simulink model "nncACCsystem_5_50"  (R2021a)
(part 4 of 14)

  "IW{2,1}(50,:)'" : Constant  Value=[0.6144727511346823600746347437961958348751068115234375;-0.6043038220130103610472360742278397083282470703125;-0.783801644557404753044238532311283051967620849609375;0.3389010522781494838540083947009406983852386474609375;-0.58015357603872319547377855997183360159397125244140625;-0.0828531218332193564179988243267871439456939697265625;0.864527016971766926189957302995026111602783203125;-0.75405004236885975199555787185090593993663787841796875;-0.924872031665473937067645238130353391170501708984375;0.2032422703217200699032929378518019802868366241455078125;-0.51577685605288647874289154060534201562404632568359375;-0.4055467735335032131160915014334022998809814453125;0.05493671254072385323752314434386789798736572265625;0.67759451705134099430694050170131959021091461181640625;-0.4116803267880932981626074251835234463214874267578125;-0.47441335981344756600464052098686806857585906982421875;-0.2043561167782945720006182455108501017093658447265625;0.82617772384643439753659777124994434416294097900390625;0.67097567185446671533810558685217984020709991455078125;0.020372107650101778375528738251887261867523193359375;0.29447303762625243184203327473369427025318145751953125;0.9440215383879964061719647361314855515956878662109375;0.6089699130967947127146544517017900943756103515625;-0.374505969506301494842404053997597657144069671630859375;-0.317174623289982360319072540733031928539276123046875;-0.6531680775410075856513003600412048399448394775390625;-0.347181889319885417233280122673022560775279998779296875;-0.410264221687952901351792434070375747978687286376953125;0.8647688276796337003560211087460629642009735107421875;0.1110609867702390118893163162283599376678466796875;-0.9109852379156795354475661952164955437183380126953125;-0.563618771772022686405989588820375502109527587890625;0.92877626827141224197248448035679757595062255859375;0.7784042806215369925126879024901427328586578369140625;0.3473576102557089928524192146142013370990753173828125;0.5260876926599216130142622205312363803386688232421875;0.87918184720997538672548898830427788197994232177734375;-0.1541856848789065204119452801023726351559162139892578125;-0.8370901964404178219325558529817499220371246337890625;-0.1124822515347916607186817827823688276112079620361328125;0.6140848728942802647878806965309195220470428466796875;-0.10539002217157571184014130949435639195144176483154296875;-0.4184943899085287188910342592862434685230255126953125;0.80793144341254274909402965931803919374942779541015625;-0.8652517508433599235928568305098451673984527587890625;0.496355196733508474693508105701766908168792724609375;0.494053866935491026168847383814863860607147216796875;-0.56814383474823326736213857657276093959808349609375;-0.226886744375101923054671715362928807735443115234375;0.90268411668282910742533431402989663183689117431640625]
      mask Display: e = 0.06;c1 = [120 150 230]/255;c2 = ([120 150 230]+0)/383;c3 = ([120 150 230]+128)/383;patch([0 1 1 0],[0 0 1 1],c1);patch([0 1 1 1-e 1-e 0+e],[0 0 1 1-e 0+e 0+e],c2);patch([0 0 1 1-e 0+e 0+e],[0 1 1 1-e 1-e 0+e],c3);plot([0 1 1 0 0],[0 0 1 1 0]);disp('weights');
  "IW{2,1}(6,:)'" : Constant  Value=[0.9179696750633585811129933063057251274585723876953125;-0.88346646120579652716742202755995094776153564453125;0.244692976834197273294790875297621823847293853759765625;-0.9438452246350792496087933614035136997699737548828125;-0.51581422348284633461190651360084302723407745361328125;0.6392679962139224958406202858895994722843170166015625;0.39256092172291989772503484346088953316211700439453125;0.1274073475641765984534004019224084913730621337890625;0.983014382423863963822441291995346546173095703125;0.21261377652534430016117994455271400511264801025390625;-0.10676266904585872408173230496686301194131374359130859375;-0.1820218409406935133887373012839816510677337646484375;-0.9638203922685992797170229096082039177417755126953125;-0.2279018435819180343759882134690997190773487091064453125;0.6813804178287572455019471817649900913238525390625;-0.2319257096428964104450898275899817235767841339111328125;1.001130044802193364006370757124386727809906005859375;-0.040503476580812568241807269942000857554376125335693359375;-0.291956084314189345807477593552903272211551666259765625;-0.6641511544489426821513688992126844823360443115234375;0.18701086129516275580186857041553594172000885009765625;0.01889726273082524554691730145350447855889797210693359375;0.488466639896083132388326930595212616026401519775390625;-0.952184047085733453741340781562030315399169921875;-0.406201797611159154399729231954552233219146728515625;0.131173827637160567149976486689411103725433349609375;0.4246658792464617082629274591454304754734039306640625;0.030614624463881780214169481268982053734362125396728515625;-0.7653854213042341481099128941423259675502777099609375;0.492109159149804853417009553595562465488910675048828125;0.275738525125877043109312580781988799571990966796875;-0.5575165603951373061164531463873572647571563720703125;-0.2552990665415426629891726406640373170375823974609375;-0.446271264888553620409084032871760427951812744140625;-0.15871405452116960077546536922454833984375;-0.280849690565660115026958010275848209857940673828125;0.49259325590821223528337213792838156223297119140625;0.484247883080110186337918776189326308667659759521484375;0.91637163929900555814356266637332737445831298828125;0.72014198242155913476381101645529270172119140625;-0.26722753351259076470824993521091528236865997314453125;0.693474476935445949266068055294454097747802734375;0.06669875991181317687050977838225662708282470703125;-0.59487481996016289276241195693728514015674591064453125;0.193733150325572200944890255414065904915332794189453125;-0.6974229533286138149605903890915215015411376953125;-0.95023164977459229074696622774354182183742523193359375;-0.1834256124171742552420028005144558846950531005859375;-0.4783530129103301664628133949008770287036895751953125;-0.70751048127678106691718085130560211837291717529296875]
      mask Display: e = 0.06;c1 = [120 150 230]/255;c2 = ([120 150 230]+0)/383;c3 = ([120 150 230]+128)/383;patch([0 1 1 0],[0 0 1 1],c1);patch([0 1 1 1-e 1-e 0+e],[0 0 1 1-e 0+e 0+e],c2);patch([0 0 1 1-e 0+e 0+e],[0 1 1 1-e 1-e 0+e],c3);plot([0 1 1 0 0],[0 0 1 1 0]);disp('weights');
  "IW{2,1}(7,:)'" : Constant  Value=[-0.980867972090291306841436380636878311634063720703125;0.78971936348265792116052352866972796618938446044921875;0.039342120990233493682541876523828250356018543243408203125;0.3719800930434804531188319742796011269092559814453125;-0.595723059500692375678454482113011181354522705078125;-0.65476188012718683495450022746808826923370361328125;0.82079906581221118155866633969708345830440521240234375;0.78456959242778889773717310163192451000213623046875;0.1931230911806987027290460900985635817050933837890625;0.488427048366413651958595210089697502553462982177734375;0.05810490529781324464675407170943799428641796112060546875;0.438775605745484131858802356873638927936553955078125;0.6583963331479651959199372868170030415058135986328125;-0.143767182260148007610922604726511053740978240966796875;0.548926493081543842578184921876527369022369384765625;-0.256575387647672237267926220738445408642292022705078125;0.50717759017805530419309434364549815654754638671875;-0.8201705525611255875872984688612632453441619873046875;-0.81636875371478268004210576691548340022563934326171875;0.547756832701655316242295157280750572681427001953125;0.226396548255365870350175327985198237001895904541015625;-0.5050091514285259819416751270182430744171142578125;-0.376156424391524690786781093265744857490062713623046875;-0.483965229362445292782268779774312861263751983642578125;0.7671583652660542984591529602766968309879302978515625;-0.66759413476073614646111309411935508251190185546875;-0.149536285868914486929526219682884402573108673095703125;0.0356486383257654804168623741134069859981536865234375;-0.5364809912488761600712905419641174376010894775390625;0.379635766555958209522714241757057607173919677734375;-0.75807806746091888072669462417252361774444580078125;-0.8879521425628060793400209149695001542568206787109375;-0.001835753065937861805423381156288087368011474609375;0.4303370024846924213335341846686787903308868408203125;0.00830634558469700579053096589632332324981689453125;-0.4866911527767816547651591463363729417324066162109375;0.9410161792518543233398986558313481509685516357421875;0.6566193894160627930745022240444086492061614990234375;0.405020058591355702759528867318294942378997802734375;0.53907900563998001342014276815461926162242889404296875;-0.04110989433774604739912916784305707551538944244384765625;0.5029607066132768533606167693505994975566864013671875;-0.8955860226761480635815360074047930538654327392578125;0.490153693698361203612279268782003782689571380615234375;0.3058058094721205488752957535325549542903900146484375;-0.4447196145408434109214113050256855785846710205078125;-0.4646406314654412117448600838542915880680084228515625;-0.8677939966654582004679241435951553285121917724609375;0.275123247728420228241930090007372200489044189453125;-0.11899464474923256152028017140764859504997730255126953125]
      mask Display: e = 0.06;c1 = [120 150 230]/255;c2 = ([120 150 230]+0)/383;c3 = ([120 150 230]+128)/383;patch([0 1 1 0],[0 0 1 1],c1);patch([0 1 1 1-e 1-e 0+e],[0 0 1 1-e 0+e 0+e],c2);patch([0 0 1 1-e 0+e 0+e],[0 1 1 1-e 1-e 0+e],c3);plot([0 1 1 0 0],[0 0 1 1 0]);disp('weights');
  "IW{2,1}(8,:)'" : Constant  Value=[-0.06407735399410119381258255089051090180873870849609375;-0.68283082031059694205765708829858340322971343994140625;-0.6603161059148481282221609944826923310756683349609375;-0.3706914380762513783196254735230468213558197021484375;-0.73915158636827260618673562930780462920665740966796875;0.73428975350198388838407481671310961246490478515625;0.95060218635651538843234220621525309979915618896484375;-0.9067290700610886045041070246952585875988006591796875;-0.8332732167303802395252887436072342097759246826171875;0.9368319573378396381002630732837133109569549560546875;0.94557012232950043983947807646472938358783721923828125;-0.170516226437212647937258225283585488796234130859375;-0.545073815603446032440615454106591641902923583984375;0.465538414095752306476327930795378051698207855224609375;-0.81784853188574135884891802561469376087188720703125;-0.1544869675737840231111164257526979781687259674072265625;0.332258729184919332499958954940666444599628448486328125;0.37661552490315608476834086104645393788814544677734375;-0.9116536259519205653845119741163216531276702880859375;-0.4143449320257059920180608969531022012233734130859375;0.1009242949167486746997468571862555108964443206787109375;0.85027929850237427000791967657278291881084442138671875;-0.305503660416293898460793343474506400525569915771484375;0.4267785913559709598530389484949409961700439453125;-0.3730091636459429427219447461538948118686676025390625;0.9594325721361993686286950833164155483245849609375;-0.94925395456621297629595801481627859175205230712890625;-0.086621871321167276391861378215253353118896484375;-0.92117713836218317879911410273052752017974853515625;-0.9749126796252569615575112038641236722469329833984375;-0.9359913347500865565820049596368335187435150146484375;0.34944472215558874950147583149373531341552734375;0.9804309399166719618534671099041588604450225830078125;-0.702038840148247356154342924128286540508270263671875;-0.4831739393233416279826997197233140468597412109375;-0.13903125857727705039224019856192171573638916015625;0.1790054588197100560176266981216031126677989959716796875;-0.28130555663841316782480816982570104300975799560546875;-0.165029675175454304536515337531454861164093017578125;0.29762772429512096561410317008267156779766082763671875;0.07987012236004879806028355915259453468024730682373046875;0.147230642125261212971309987551649101078510284423828125;-0.59547301053531764836179718258790671825408935546875;-0.314192711422670967191805857510189525783061981201171875;-0.10479329307725386566385594733219477348029613494873046875;-0.494784453168344295903580132289789617061614990234375;0.84635061232047592572058647419908083975315093994140625;0.6462217446144540300423386725015006959438323974609375;-0.753402215742656977681690477766096591949462890625;-0.51731503262576661317240223070257343351840972900390625]
      mask Display: e = 0.06;c1 = [120 150 230]/255;c2 = ([120 150 230]+0)/383;c3 = ([120 150 230]+128)/383;patch([0 1 1 0],[0 0 1 1],c1);patch([0 1 1 1-e 1-e 0+e],[0 0 1 1-e 0+e 0+e],c2);patch([0 0 1 1-e 0+e 0+e],[0 1 1 1-e 1-e 0+e],c3);plot([0 1 1 0 0],[0 0 1 1 0]);disp('weights');
  "IW{2,1}(9,:)'" : Constant  Value=[-0.102714725663822559198479211772792041301727294921875;0.4368170165488063361181048094294965267181396484375;-0.51179821386116230996776721440255641937255859375;-0.787132888983194778376173417200334370136260986328125;-0.6590563544371967896751129956101067364215850830078125;0.0784485917003274746406304984702728688716888427734375;-0.7862631079594495364659678671159781515598297119140625;0.805272154985862353981929118162952363491058349609375;-0.4183870521965247224471795561839826405048370361328125;0.2439889456538122392004197536152787506580352783203125;-0.501606876311778027144328007125295698642730712890625;0.8303594512562797458343766265898011624813079833984375;-0.2557645626674929228983046414214186370372772216796875;0.0319540177471291375610462637268938124179840087890625;-0.6444998703933177974789714426151476800441741943359375;0.3866189078107942211914860308752395212650299072265625;0.91232573693869856157334652380086481571197509765625;0.571427116455696992858293015160597860813140869140625;-0.9689301839636759172691427011159248650074005126953125;-0.2074717539773345276188365460257045924663543701171875;0.4953012002888812492784609275986440479755401611328125;-0.2659602519525348096607331171981059014797210693359375;0.1714702338959359639858348600682802498340606689453125;0.449448527641817197064710853737778961658477783203125;0.7469316764358662208422856565448455512523651123046875;-0.04222883079584160981312379590235650539398193359375;0.960848497813605373352174865431152284145355224609375;0.8105326403854800076942410669289529323577880859375;0.4344707041244746381636332444031722843647003173828125;0.0714152851764093821174128606799058616161346435546875;-0.331011733793374229861683488707058131694793701171875;0.0242470574157973572937407880090177059173583984375;-0.60912441145073170645218851859681308269500732421875;-0.1507646675101452782286060028127394616603851318359375;0.9280407269415540394419394942815415561199188232421875;0.1478420865894018998432102307560853660106658935546875;0.572746574072698688695481905597262084484100341796875;-0.80497354396350839778051522444002330303192138671875;0.6750655125951308122012051171623170375823974609375;-0.2406190148984588272895734917256049811840057373046875;0.0853845073917802732665904841269366443157196044921875;-0.0019238695503458469460156265995465219020843505859375;-0.359935279909433969436349798343144357204437255859375;-0.5085445449720047417230261999065987765789031982421875;-0.662466683688774704563684281310997903347015380859375;-0.622816308705548937751927951467223465442657470703125;0.782043018155911706656979731633327901363372802734375;0.3763126465426847033768353867344558238983154296875;0.814751469791895832628370044403709471225738525390625;-0.3952772922938365685041617325623519718647003173828125]
      mask Display: e = 0.06;c1 = [120 150 230]/255;c2 = ([120 150 230]+0)/383;c3 = ([120 150 230]+128)/383;patch([0 1 1 0],[0 0 1 1],c1);patch([0 1 1 1-e 1-e 0+e],[0 0 1 1-e 0+e 0+e],c2);patch([0 0 1 1-e 0+e 0+e],[0 1 1 1-e 1-e 0+e],c3);plot([0 1 1 0 0],[0 0 1 1 0]);disp('weights');
  Mux : Mux  Inputs=50
      mask Display: e = 0.06;c1 = [120 150 230]/255;c2 = ([120 150 230]+0)/383;c3 = ([120 150 230]+128)/383;patch([0 1 1 0],[0 0 1 1],c1);patch([0 1 1 1-e 1-e 0+e],[0 0 1 1-e 0+e 0+e],c2);patch([0 0 1 1-e 0+e 0+e],[0 1 1 1-e 1-e 0+e],c3);plot([0 1 1 0 0],[0 0 1 1 0]);disp('Mux');
  dotprod{1..50} (50 alike) : neural/Weight Functions/dotprod
  "lz{2,1}" : Outport
      mask Display: e = 0.06;c1 = [120 230 180]/255;c2 = ([120 230 180]+0)/(256+128);c3 = ([120 230 180]+128)/(256+128);patch([0 1 1 0],[0 0 1 1],c1);patch([0 1 1 1-e 1-e 0+e],[0 0 1 1-e 0+e 0+e],c2);patch([0 0 1 1-e 0+e 0+e],[0 1 1 1-e 1-e 0+e],c3);plot([0 1 1 0 0],[0 0 1 1 0]);
  wires:
  Mux/1 -> "lz{2,1}"/1
  dotprod50/1 -> Mux/50
  "IW{2,1}(50,:)'"/1 -> dotprod50/1
  dotprod49/1 -> Mux/49
  "IW{2,1}(49,:)'"/1 -> dotprod49/1
  dotprod48/1 -> Mux/48
  "IW{2,1}(48,:)'"/1 -> dotprod48/1
  dotprod47/1 -> Mux/47
  "IW{2,1}(47,:)'"/1 -> dotprod47/1
  dotprod46/1 -> Mux/46
  "IW{2,1}(46,:)'"/1 -> dotprod46/1
  dotprod45/1 -> Mux/45
  "IW{2,1}(45,:)'"/1 -> dotprod45/1
  dotprod44/1 -> Mux/44
  "IW{2,1}(44,:)'"/1 -> dotprod44/1
  dotprod43/1 -> Mux/43
  "IW{2,1}(43,:)'"/1 -> dotprod43/1
  dotprod42/1 -> Mux/42
  "IW{2,1}(42,:)'"/1 -> dotprod42/1
  dotprod41/1 -> Mux/41
  "IW{2,1}(41,:)'"/1 -> dotprod41/1
  dotprod40/1 -> Mux/40
  "IW{2,1}(40,:)'"/1 -> dotprod40/1
  dotprod39/1 -> Mux/39
  "IW{2,1}(39,:)'"/1 -> dotprod39/1
  dotprod38/1 -> Mux/38
  "IW{2,1}(38,:)'"/1 -> dotprod38/1
  dotprod37/1 -> Mux/37
  "IW{2,1}(37,:)'"/1 -> dotprod37/1
  dotprod36/1 -> Mux/36
  "IW{2,1}(36,:)'"/1 -> dotprod36/1
  dotprod35/1 -> Mux/35
  "IW{2,1}(35,:)'"/1 -> dotprod35/1
  dotprod34/1 -> Mux/34
  "IW{2,1}(34,:)'"/1 -> dotprod34/1
  dotprod33/1 -> Mux/33
  "IW{2,1}(33,:)'"/1 -> dotprod33/1
  dotprod32/1 -> Mux/32
  "IW{2,1}(32,:)'"/1 -> dotprod32/1
  dotprod31/1 -> Mux/31
  "IW{2,1}(31,:)'"/1 -> dotprod31/1
  dotprod30/1 -> Mux/30
  "IW{2,1}(30,:)'"/1 -> dotprod30/1
  dotprod29/1 -> Mux/29
  "IW{2,1}(29,:)'"/1 -> dotprod29/1
  dotprod28/1 -> Mux/28
  "IW{2,1}(28,:)'"/1 -> dotprod28/1
  dotprod27/1 -> Mux/27
  "IW{2,1}(27,:)'"/1 -> dotprod27/1
  dotprod26/1 -> Mux/26
  "IW{2,1}(26,:)'"/1 -> dotprod26/1
  dotprod25/1 -> Mux/25
  "IW{2,1}(25,:)'"/1 -> dotprod25/1
  dotprod24/1 -> Mux/24
  "IW{2,1}(24,:)'"/1 -> dotprod24/1
  dotprod23/1 -> Mux/23
  "IW{2,1}(23,:)'"/1 -> dotprod23/1
  dotprod22/1 -> Mux/22
  "IW{2,1}(22,:)'"/1 -> dotprod22/1
  dotprod21/1 -> Mux/21
  "IW{2,1}(21,:)'"/1 -> dotprod21/1
  dotprod20/1 -> Mux/20
  "IW{2,1}(20,:)'"/1 -> dotprod20/1
  dotprod19/1 -> Mux/19
  "IW{2,1}(19,:)'"/1 -> dotprod19/1
  dotprod18/1 -> Mux/18
  "IW{2,1}(18,:)'"/1 -> dotprod18/1
  dotprod17/1 -> Mux/17
  "IW{2,1}(17,:)'"/1 -> dotprod17/1
  dotprod16/1 -> Mux/16
  "IW{2,1}(16,:)'"/1 -> dotprod16/1
  dotprod15/1 -> Mux/15
  "IW{2,1}(15,:)'"/1 -> dotprod15/1
  dotprod14/1 -> Mux/14
  "IW{2,1}(14,:)'"/1 -> dotprod14/1
  dotprod13/1 -> Mux/13
  "IW{2,1}(13,:)'"/1 -> dotprod13/1
  dotprod12/1 -> Mux/12
  "IW{2,1}(12,:)'"/1 -> dotprod12/1
  dotprod11/1 -> Mux/11
  "IW{2,1}(11,:)'"/1 -> dotprod11/1
  dotprod10/1 -> Mux/10
  "IW{2,1}(10,:)'"/1 -> dotprod10/1
  dotprod9/1 -> Mux/9
  "IW{2,1}(9,:)'"/1 -> dotprod9/1
  dotprod8/1 -> Mux/8
  "IW{2,1}(8,:)'"/1 -> dotprod8/1
  dotprod7/1 -> Mux/7
  "IW{2,1}(7,:)'"/1 -> dotprod7/1
  dotprod6/1 -> Mux/6
  "IW{2,1}(6,:)'"/1 -> dotprod6/1
  dotprod5/1 -> Mux/5
  "IW{2,1}(5,:)'"/1 -> dotprod5/1
  dotprod4/1 -> Mux/4
  "IW{2,1}(4,:)'"/1 -> dotprod4/1
  dotprod3/1 -> Mux/3
  "IW{2,1}(3,:)'"/1 -> dotprod3/1
  dotprod2/1 -> Mux/2
  "IW{2,1}(2,:)'"/1 -> dotprod2/1
  dotprod1/1 -> Mux/1
  "ad{2,1}"/1 -> dotprod50/2, dotprod49/2, dotprod48/2, dotprod47/2, dotprod46/2, dotprod45/2, dotprod44/2, dotprod43/2, dotprod42/2, dotprod41/2, dotprod40/2, dotprod39/2, dotprod38/2, dotprod37/2, dotprod36/2, dotprod35/2, dotprod34/2, dotprod33/2, dotprod32/2, dotprod31/2, dotprod30/2, dotprod29/2, dotprod28/2, dotprod27/2, dotprod26/2, dotprod25/2, dotprod24/2, dotprod23/2, dotprod22/2, dotprod21/2, dotprod20/2, dotprod19/2, dotprod18/2, dotprod17/2, dotprod16/2, dotprod15/2, dotprod14/2, dotprod13/2, dotprod12/2, dotprod11/2, dotprod10/2, dotprod9/2, dotprod8/2, dotprod7/2, dotprod6/2, dotprod5/2, dotprod4/2, dotprod3/2, dotprod2/2, dotprod1/2
  "IW{2,1}(1,:)'"/1 -> dotprod1/1
